simulink model "controller"  (Simulink 8.0)
settings: Solver=FixedStepDiscrete  StartTime=0.0  StopTime=inf  FixedStep=Ts  RelTol=1e-3
InitFcn:
  | initTorqueBalancing;
values from neighbouring files (symbols this model uses):
  DT = 30    [initRov14.m]
  kImp = [kImpTorso,kImpArms,kImpArms,kImpLegs,kImpLegs]    [initRov14.m]
  qFin = -ones(25,1)*5    [initRov14.m]
  Rf = [R, zeros(3,3); zeros(3,3), R]    [initRov14.m]    (also in initSharedMem_Nori.m)
undefined symbols (not defined in the file or in its folder): DiscIntNeverNeededParam, kH, states
libraries: WBCLibrary x27, simulink x2, dspsigops x2
settings Model: Creator=daniele  LastModifiedBy=daniele
settings DebuggingCC: FcnCallInpInsideContextMsg=EnableAllAsWarning
settings GRTTargetCC: CombineOutputUpdateFcns=off  GRTInterface=on

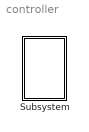
== system controller ==
  Subsystem : Subsystem  mask{robotName='iCubGenova01', Ts=0.01, localName='dynamicBalancing'}
      mask prompts: robotName "robot name"; localName "module name"

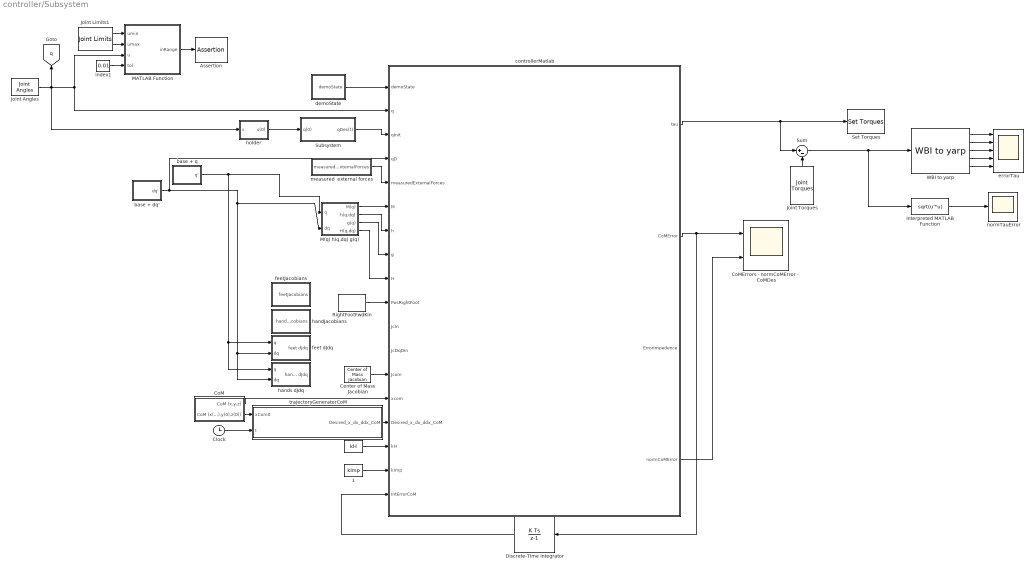
== system controller/Subsystem ==
  "    " : Constant  Value=kH
  "    1" : Constant  Value=kImp
  Assertion : Assertion  Enabled=on
  Center of Mass Jacobian : WBCLibrary/wholeBodyModel/Jacobians/Center of Mass Jacobian  robotName=robotName  localName=localName
  Clock : Clock
  "CoM " : Subsystem
  "CoMErrors - normCoMError -   CoMDes " : Scope  NumInputPorts=2
      settings: ShowLegends=on  TimeRange=35  YMin=-0.1~0  YMax=0.04000000000000001~0.007  SaveName=CoMErrors
  Discrete-Time Integrator : DiscreteIntegrator  InitialCondition=[0 0 0]  SampleTime=Ts  ICPrevOutput=DiscIntNeverNeededParam  ICPrevScaledInput=DiscIntNeverNeededParam
  Interpreted MATLAB Function : MATLABFcn  MATLABFcn=sqrt(u'*u)
  Joint Angles : WBCLibrary/wholeBodyStates/Joint Angles  robotName=robotName  localName=localName
  Joint Limits1 : WBCLibrary/wholeBodyModel/Joint Limits  robotName=robotName  localName=localName
  Joint Torques : WBCLibrary/wholeBodyStates/Joint Torques  robotName=robotName  localName=localName
  M(q) h(q,dq) g(q) : Subsystem
  MATLAB Function : MATLAB Function  TreatAsAtomicUnit=on
  RightFootFwdKin : WBCLibrary/wholeBodyModel/Forward Kinematics/RightFootFwdKin  robotName=robotName  localName=localName
  Set Torques : WBCLibrary/wholeBodyActuators/Set Torques  val=6  robotName=robotName  localName=localName
  Subsystem : Subsystem
  Sum : Sum  Inputs=|+-
  WBI to yarp : WBCLibrary/Utilities/WBI to yarp
  base + dq' : Subsystem
  base + q : Subsystem
  controllerMatlab : MATLAB Function  TreatAsAtomicUnit=on
  demoState : Subsystem
  errorTau : Scope  NumInputPorts=5
      settings: TimeRange=20  YMin=-12~-5~-5~-5~-5  YMax=6~5~5~5~5
  feet dJdq : Subsystem
  feetJacobians : Subsystem
  handJacobians : Subsystem
  hands dJdq : Subsystem
  holder : Subsystem
  index1 : Constant  Value=0.01  VectorParams1D=off
  measured  external forces : Subsystem
  normTauError : Scope
      settings: TimeRange=80  YMin=0  YMax=60  SaveName=normTauError
  trajectoryGeneratorCoM : MATLAB Function  TreatAsAtomicUnit=on
  tag scope: q=global
  wires:
  Center of Mass Jacobian/1 -> controllerMatlab/13(Jcom)
  "    "/1 -> controllerMatlab/16(kH)
  trajectoryGeneratorCoM/1(Desired_x_dx_ddx_CoM) -> controllerMatlab/15(Desired_x_dx_ddx_CoM)
  Clock/1 -> trajectoryGeneratorCoM/2(t)
  "CoM "/2(CoM (x(0),y(0),z(0))) -> trajectoryGeneratorCoM/1(xCom0)
  holder/1(s(0)) -> Subsystem/1(q(0))
  RightFootFwdKin/1 -> controllerMatlab/10(PosRightFoot)
  Discrete-Time Integrator/1 -> controllerMatlab/18(IntErrorCoM)
  base + q/1(q') -> hands dJdq/1(q), feet dJdq/1(q), M(q) h(q,dq) g(q)/1(q)
  base + dq'/1(dq') -> controllerMatlab/4(qD), hands dJdq/2(dq), feet dJdq/2(dq), M(q) h(q,dq) g(q)/2(dq)
  Joint Limits1/1 -> MATLAB Function/1(umin)
  Joint Limits1/2 -> MATLAB Function/2(umax)
  Joint Angles/1 -> [q], MATLAB Function/3(u), controllerMatlab/2(q), holder/1(s)
  index1/1 -> MATLAB Function/4(tol)
  controllerMatlab/2(CoMError) -> Discrete-Time Integrator/1, "CoMErrors - normCoMError -   CoMDes "/1
  controllerMatlab/4(normCoMError) -> "CoMErrors - normCoMError -   CoMDes "/2
  "    1"/1 -> controllerMatlab/17(kImp)
  MATLAB Function/1(inRange) -> Assertion/1
  measured  external forces/1(measuredExternalForces) -> controllerMatlab/5(measuredExternalForces)
  controllerMatlab/1(tau) -> Sum/1, Set Torques/1
  Joint Torques/1 -> Sum/2
  Interpreted MATLAB Function/1 -> normTauError/1
  Sum/1 -> WBI to yarp/1, Interpreted MATLAB Function/1
  WBI to yarp/1 -> errorTau/1
  WBI to yarp/2 -> errorTau/2
  WBI to yarp/3 -> errorTau/3
  WBI to yarp/4 -> errorTau/4
  WBI to yarp/5 -> errorTau/5
  Subsystem/1(qDes(t)) -> controllerMatlab/3(qInit)
  M(q) h(q,dq) g(q)/1(M(q)) -> controllerMatlab/6(M)
  M(q) h(q,dq) g(q)/2(h(q,dq)) -> controllerMatlab/7(h)
  M(q) h(q,dq) g(q)/3(g(q)) -> controllerMatlab/8(g)
  "CoM "/1(CoM (x,y,z)) -> controllerMatlab/14(xcom)
  M(q) h(q,dq) g(q)/4(H(q,dq)) -> controllerMatlab/9(H)
  demoState/1(demoState) -> controllerMatlab/1(demoState)

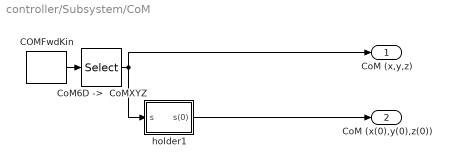
== system controller/Subsystem/CoM  ==
  "COMFwdKin " : WBCLibrary/wholeBodyModel/Forward Kinematics/COMFwdKin   robotName=robotName  localName=localName
  "CoM6D ->  CoMXYZ" : Selector  InputPortWidth=7  IndexOptions=Index vector (dialog)  Indices=[1 2 3]  OutputSizes=1
  holder1 : Subsystem
  CoM (x,y,z) : Outport
  CoM (x(0),y(0),z(0)) : Outport  Port=2
  wires:
  "COMFwdKin "/1 -> "CoM6D ->  CoMXYZ"/1
  "CoM6D ->  CoMXYZ"/1 -> holder1/1(s), CoM (x,y,z)/1
  holder1/1(s(0)) -> CoM (x(0),y(0),z(0))/1

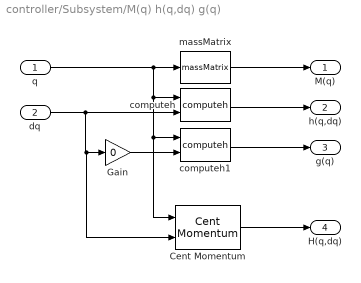
== system controller/Subsystem/M(q) h(q,dq) g(q) ==
  q : Inport
  dq : Inport  Port=2
  Cent Momentum : WBCLibrary/wholeBodyModel/Dynamics/Cent Momentum  robotName=robotName  localName=localName
  Gain : Gain  Gain=0
  computeh : WBCLibrary/wholeBodyModel/Dynamics/computeh  val=7  robotname=robotName  localname=localName
  computeh1 : WBCLibrary/wholeBodyModel/Dynamics/computeh  val=7  robotname=robotName  localname=localName
  massMatrix : WBCLibrary/wholeBodyModel/Dynamics/massMatrix  val=8  robotname=robotName  localname=localName
  M(q) : Outport
  h(q,dq) : Outport  Port=2
  g(q) : Outport  Port=3
  H(q,dq) : Outport  Port=4
  wires:
  Gain/1 -> computeh1/2
  computeh1/1 -> g(q)/1
  computeh/1 -> h(q,dq)/1
  massMatrix/1 -> M(q)/1
  q/1 -> Cent Momentum/1, computeh1/1, computeh/1, massMatrix/1
  dq/1 -> Cent Momentum/2, Gain/1, computeh/2
  Cent Momentum/1 -> H(q,dq)/1

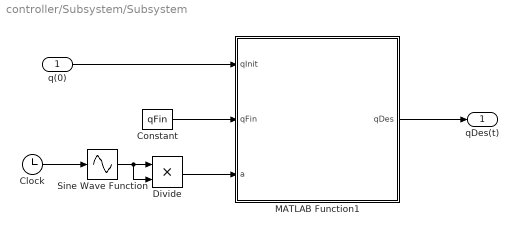
== system controller/Subsystem/Subsystem ==
  q(0) : Inport
  Clock : Clock
  Constant : Constant  Value=qFin
  Divide : Product  Inputs=**
  MATLAB Function1 : MATLAB Function  TreatAsAtomicUnit=on
  Sine Wave Function : Sin  TimeSource=Use external signal  Frequency=pi/DT  SampleTime=0
  qDes(t) : Outport
  wires:
  q(0)/1 -> MATLAB Function1/1(qInit)
  MATLAB Function1/1(qDes) -> qDes(t)/1
  Constant/1 -> MATLAB Function1/2(qFin)
  Clock/1 -> Sine Wave Function/1
  Sine Wave Function/1 -> Divide/2, Divide/1
  Divide/1 -> MATLAB Function1/3(a)

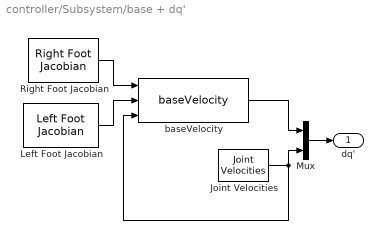
== system controller/Subsystem/base + dq' ==
  Joint Velocities : WBCLibrary/wholeBodyStates/Joint Velocities  robotName=robotName  localName=localName
  Left Foot Jacobian : WBCLibrary/wholeBodyModel/Jacobians/Left Foot Jacobian  robotName=robotName  localName=localName
  Mux : Mux  Inputs=2
  Right Foot Jacobian : WBCLibrary/wholeBodyModel/Jacobians/Right Foot Jacobian  robotName=robotName  localName=localName
  baseVelocity : WBCLibrary/Utilities/baseVelocity
  dq' : Outport
  wires:
  Left Foot Jacobian/1 -> baseVelocity/2
  Right Foot Jacobian/1 -> baseVelocity/1
  baseVelocity/1 -> Mux/1
  Joint Velocities/1 -> baseVelocity/3, Mux/2
  Mux/1 -> dq'/1

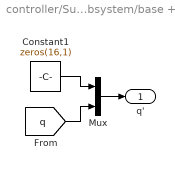
== system controller/Subsystem/base + q ==
  Constant1 : Constant  Value=zeros(16,1)
  Mux : Mux  Inputs=2
  q' : Outport
  wires:
  Mux/1 -> q'/1
  [q] -> Mux/2
  Constant1/1 -> Mux/1

== system controller/Subsystem/demoState ==
  "    3" : Constant  Value=states
  MATLAB Function1 : MATLAB Function  TreatAsAtomicUnit=on
  Reading the demo  state as sent from lua : WBCLibrary/Utilities/yarp read  from='/wholeBodyDyanmicsTree/right_leg/endEffectorWrench:o'  to='...'  num=1
  demoState : Outport
  wires:
  MATLAB Function1/1(stateOut) -> demoState/1
  "    3"/1 -> MATLAB Function1/2(states)
  Reading the demo  state as sent from lua/1 -> MATLAB Function1/1(stateIn)

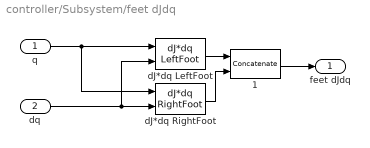
== system controller/Subsystem/feet dJdq ==
  q : Inport
  dq : Inport  Port=2
  " 1" : Concatenate  Mode=Multidimensional array
  dJ*dq LeftFoot : WBCLibrary/wholeBodyModel/Dynamics/dJ*dq LeftFoot  val=9  robotName=robotName  localName=localName
  dJ*dq RightFoot : WBCLibrary/wholeBodyModel/Dynamics/dJ*dq RightFoot  val=9  robotName=robotName  localName=localName
  feet dJdq : Outport
  wires:
  dJ*dq LeftFoot/1 -> " 1"/1
  dJ*dq RightFoot/1 -> " 1"/2
  " 1"/1 -> feet dJdq/1
  q/1 -> dJ*dq RightFoot/1, dJ*dq LeftFoot/1
  dq/1 -> dJ*dq LeftFoot/2, dJ*dq RightFoot/2

== system controller/Subsystem/feetJacobians ==
  " " : Concatenate  Mode=Multidimensional array
  Left Foot Jacobian : WBCLibrary/wholeBodyModel/Jacobians/Left Foot Jacobian  robotName=robotName  localName=localName
  Right Foot Jacobian : WBCLibrary/wholeBodyModel/Jacobians/Right Foot Jacobian  robotName=robotName  localName=localName
  feetJacobians : Outport
  wires:
  Left Foot Jacobian/1 -> " "/1
  Right Foot Jacobian/1 -> " "/2
  " "/1 -> feetJacobians/1

== system controller/Subsystem/handJacobians ==
  " " : Concatenate  Mode=Multidimensional array
  Left Hand Jacobian : WBCLibrary/wholeBodyModel/Jacobians/Left Hand Jacobian  robotName=robotName  localName=localName
  Right Hand Jacobian : WBCLibrary/wholeBodyModel/Jacobians/Right Hand Jacobian  robotName=robotName  localName=localName
  handJacobians : Outport
  wires:
  " "/1 -> handJacobians/1
  Left Hand Jacobian/1 -> " "/1
  Right Hand Jacobian/1 -> " "/2

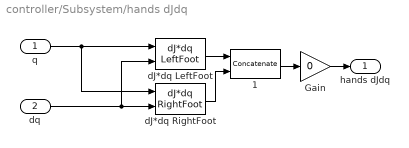
== system controller/Subsystem/hands dJdq ==
  q : Inport
  dq : Inport  Port=2
  " 1" : Concatenate  Mode=Multidimensional array
  Gain : Gain  Gain=0
  dJ*dq LeftFoot : WBCLibrary/wholeBodyModel/Dynamics/dJ*dq LeftFoot  val=9  robotName=robotName  localName=localName
  dJ*dq RightFoot : WBCLibrary/wholeBodyModel/Dynamics/dJ*dq RightFoot  val=9  robotName=robotName  localName=localName
  hands dJdq : Outport
  wires:
  dJ*dq LeftFoot/1 -> " 1"/1
  dJ*dq RightFoot/1 -> " 1"/2
  " 1"/1 -> Gain/1
  q/1 -> dJ*dq RightFoot/1, dJ*dq LeftFoot/1
  dq/1 -> dJ*dq LeftFoot/2, dJ*dq RightFoot/2
  Gain/1 -> hands dJdq/1

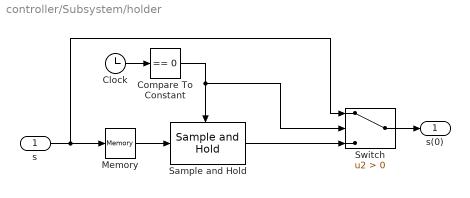
== system controller/Subsystem/holder ==
  s : Inport
  Clock : Clock
  Compare To Constant : simulink/Logic and Bit Operations/Compare To Constant  relop===  const=0  OutDataTypeStr=boolean
  Memory : Memory
  Sample and Hold : dspsigops/Sample and Hold  trig=Falling edge  initCond=0  latchinput=off
  Switch : Switch  Criteria=u2 > Threshold
  s(0) : Outport
  wires:
  s/1 -> Switch/1, Memory/1
  Clock/1 -> Compare To Constant/1
  Compare To Constant/1 -> Sample and Hold/Trigger, Switch/2
  Sample and Hold/1 -> Switch/3
  Switch/1 -> s(0)/1
  Memory/1 -> Sample and Hold/1

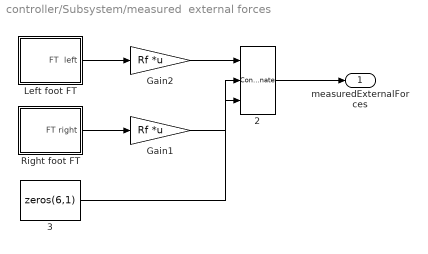
== system controller/Subsystem/measured  external forces ==
  "    3" : Constant  Value=zeros(6,1)
  " 2" : Concatenate  NumInputs=3  Mode=Multidimensional array
  Gain1 : Gain  Gain=Rf  Multiplication=Matrix(K*u)
  Gain2 : Gain  Gain=Rf  Multiplication=Matrix(K*u)
  Left foot FT : Subsystem
  Right foot FT : Subsystem
  measuredExternalForces : Outport
  wires:
  Right foot FT/1(FT right) -> Gain1/1
  Left foot FT/1(FT  left) -> Gain2/1
  Gain2/1 -> " 2"/1
  Gain1/1 -> " 2"/2
  "    3"/1 -> " 2"/3
  " 2"/1 -> measuredExternalForces/1

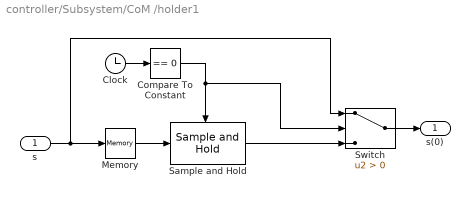
== system controller/Subsystem/CoM /holder1 ==
  s : Inport
  Clock : Clock
  Compare To Constant : simulink/Logic and Bit Operations/Compare To Constant  relop===  const=0  OutDataTypeStr=boolean
  Memory : Memory
  Sample and Hold : dspsigops/Sample and Hold  trig=Falling edge  initCond=0  latchinput=off
  Switch : Switch  Criteria=u2 > Threshold
  s(0) : Outport
  wires:
  s/1 -> Switch/1, Memory/1
  Clock/1 -> Compare To Constant/1
  Compare To Constant/1 -> Sample and Hold/Trigger, Switch/2
  Sample and Hold/1 -> Switch/3
  Switch/1 -> s(0)/1
  Memory/1 -> Sample and Hold/1

== system controller/Subsystem/measured  external forces/Left foot FT ==
  Mux : Mux  Inputs=6
  yarp read : WBCLibrary/Utilities/yarp read  from='/wholeBodyDyanmicsTree/left_leg/endEffectorWrench:o'  to='...'  num=6
  FT  left : Outport
  wires:
  yarp read/1 -> Mux/1
  yarp read/2 -> Mux/2
  yarp read/3 -> Mux/3
  yarp read/4 -> Mux/4
  yarp read/5 -> Mux/5
  yarp read/6 -> Mux/6
  Mux/1 -> FT  left/1

== system controller/Subsystem/measured  external forces/Right foot FT ==
  Mux : Mux  Inputs=6
  yarp read : WBCLibrary/Utilities/yarp read  from='/wholeBodyDyanmicsTree/right_leg/endEffectorWrench:o'  to='...'  num=6
  FT right : Outport
  wires:
  yarp read/1 -> Mux/1
  yarp read/2 -> Mux/2
  yarp read/3 -> Mux/3
  yarp read/4 -> Mux/4
  yarp read/5 -> Mux/5
  yarp read/6 -> Mux/6
  Mux/1 -> FT right/1

== matlab function Subsystem/trajectoryGeneratorCoM ==
  data: Desired_x_dx_ddx_CoM output double; xCom0 input double; t input double
function Desired_x_dx_ddx_CoM = fcn(xCom0,t)
%#codegen

e3 = [0;1;0];
A = 0.015;
f = 0.15;

xcomDes    = xCom0 + A*sin(2*pi*f*t)*e3;
% xcomDes(3) =  xcomDes(3) + 0.01;
xDcomDes   =         A*2*pi*f*cos(2*pi*f*t)*e3;
xDDcomDes  =        -A*(2*pi*f)^2*sin(2*pi*f*t)*e3;

Desired_x_dx_ddx_CoM = [xcomDes,xDcomDes,xDDcomDes];

== matlab function Subsystem/controllerMatlab ==
  data: demoState input double; q input double; qInit input double; qD input double; measuredExternalForces input double; M input double; h input double; g input double; H input double; PosRightFoot input double; JcIn input double; JcDqDIn input double; tau output double; Jcom input double; xcom input double; Desired_x_dx_ddx_CoM input double; kH input double; kImp input double; CoMError output double; IntErrorCoM input double; ErrorImpedence output double; normCoMError output double
function [tau,CoMError,ErrorImpedence,normCoMError] = fcn(demoState,q,qInit,qD, measuredExternalForces, M, h, g, H, PosRightFoot, JcIn, JcDqDIn, Jcom, xcom, Desired_x_dx_ddx_CoM, kH, kImp, IntErrorCoM)
%#codegen

PINV_TOL = 1e-5;
gravAcc        = 9.81;

n = 25;
St    = [zeros(6,n);eye(n,n)];

m     = M(1,1);
grav = [zeros(2,1);-m*gravAcc;zeros(3,1)];

% Definition of reference accelerations for CoM and Joints that ensure
% stabilization of desired trajectories xDcomDes and qDes 

xDcom      = Jcom(1:3,:)*qD;
xDDcomStar = Desired_x_dx_ddx_CoM(:,3) - kH(1)*(xcom - Desired_x_dx_ddx_CoM(:,1)) - kH(2)*IntErrorCoM - kH(3)*(xDcom - Desired_x_dx_ddx_CoM(:,2));

Pr =  PosRightFoot(1:3) - xcom; % Application point of the contact force on the right foot w.r.t. CoM

A  = [ eye(3),   zeros(3),eye(3), zeros(3);
      -Sf(xcom),  eye(3), Sf(Pr), eye(3) ];
hwDotDes = H(4:end);
hDotDes  = [ m*xDDcomStar ;
             -kH(4)*hwDotDes  ]; 
Jc = JcIn;         
JcDqD = JcDqDIn;

FeetMeasuredWrenches   = measuredExternalForces(1:12);
LeftHandMeasuredForce  = measuredExternalForces(13:15);
RightHandMeasuredForce = measuredExternalForces(16:18);


pinvA = pinv(A, PINV_TOL);
fd    = pinvA*(hDotDes-grav) ;% + (eye(length(fextMeas)) - pinvA*A)*fextMeas;

Minv = inv(M);
JcMinv        = Jc*Minv;
PInv_JcMinvSt = pinv(JcMinv*St, PINV_TOL);
N0            = eye(n) - PInv_JcMinvSt*JcMinv*St;

FeetMeasuredWrenches = fd;

tau1 = PInv_JcMinvSt*(JcMinv*h - JcDqD - JcMinv*Jc'*fd);
LinearizedDynamics = g(7:end)-Jc(:,7:end)'*FeetMeasuredWrenches - kImp.*(q-qInit);% - tau1 -diag(kDam)*N0'*qD(7:end) ;  %-kDam.*qD(7:end) 

tau0 = LinearizedDynamics;

tau = tau1 + N0*tau0;

% f = (JcMinv*Jc')^-1*(JcMinv*(h-[zeros(6,1);tau])-JcDqD);

CoMError    = xcom - xcomDes;
normCoMError  = norm(CoMError);
ErrorImpedence   = tau + LinearizedDynamics;

== matlab function Subsystem/Subsystem/MATLAB Function1 ==
  data: qInit input double; qFin input double; qDes output double; a input double
function qDes = checkRange(qInit,qFin,a)
%#codegen
 
qFin(qFin == -5) = qInit(qFin == -5);

qDes = qInit + a*(qFin-qInit);

== matlab function Subsystem/MATLAB Function ==
  data: umin input double; umax input double; u input double; inRange output double; tol input double
function inRange = checkRange(umin, umax, u, tol)
%#codegen

res = u < umin + tol | u > umax - tol;
res = sum(res);
if res==0
    inRange = 1;
else
    inRange = 0;
    u < umin + tol | u > umax - tol
end

== matlab function Subsystem/demoState/MATLAB Function1 ==
  data: stateIn input double; stateOut output double; states input double
function stateOut = checkRange(stateIn,states)
%#codegen
 
if stateIn == states(1)
    stateOut = 'balanceNoHandContact';
end

if stateIn == states(2)
    stateOut = 'balanceAndSeekContacts';
end

if stateIn == states(3)
    stateOut = 'leftHandInContact_rightHandSeeks_keepBalance';
end

if stateIn == states(4)
    stateOut = 'rightHandInContact_leftHandSeeks_keepBalance';
end

if stateIn == states(5)
    stateOut = 'bothHandsInContact_balance'; 
end
